simulink model "PI_controller_antiwindup1"  (R2019b)
settings: Solver=FixedStepAuto  StartTime=0.0  StopTime=15  FixedStep=0.005  RelTol=1e-3
settings Model: Creator=suvo  LastModifiedBy=suvo

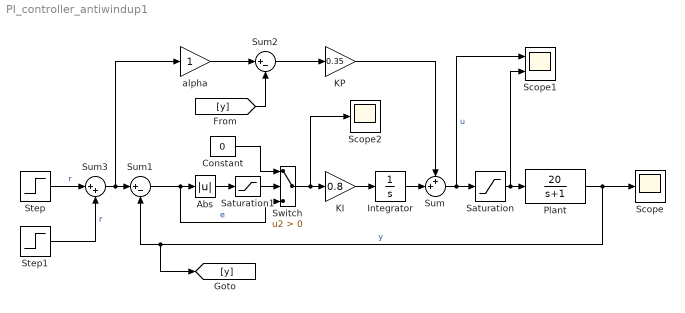
== system PI_controller_antiwindup1 ==
  Abs : Abs
  Constant : Constant  Value=0
  Integrator : Integrator
  KI : Gain  Gain=0.8
  KP : Gain  Gain=0.35
  Plant : TransferFcn  Numerator=20  Denominator=[1 1]
  Saturation : Saturate  UpperLimit=0.03  LowerLimit=-.03
  Saturation1 : Saturate
  Scope : Scope
  Scope1 : Scope  NumInputPorts=2
  Scope2 : Scope
  Step : Step  SampleTime=0
  Step1 : Step  Time=5  After=-1  SampleTime=0
  Sum : Sum  Inputs=++|
  Sum1 : Sum  Inputs=|+-
  Sum2 : Sum  Inputs=|+-
  Sum3 : Sum  Inputs=|++
  Switch : Switch  Criteria=u2 > Threshold
  alpha : Gain
  wires:
  KI/1 -> Integrator/1
  Plant/1 -> Scope/1, [y], Sum1/2  "y"
  Sum2/1 -> KP/1
  KP/1 -> Sum/1
  Integrator/1 -> Sum/2
  Sum/1 -> Scope1/1, Saturation/1  "u"
  [y] -> Sum2/2
  alpha/1 -> Sum2/1
  Saturation/1 -> Scope1/2, Plant/1
  Step/1 -> Sum3/1  "r"
  Sum3/1 -> alpha/1, Sum1/1
  Step1/1 -> Sum3/2  "r"
  Constant/1 -> Switch/1
  Switch/1 -> Scope2/1, KI/1
  Sum1/1 -> Switch/3, Abs/1  "e"
  Abs/1 -> Saturation1/1
  Saturation1/1 -> Switch/2
